simulink model "ControlLoopSim"  (R2018b)
settings: Solver=FixedStepAuto  StartTime=0.0  StopTime=Tsim  FixedStep=Ts  RelTol=1e-3
values from neighbouring files (symbols this model uses):
  Ts = 0.01    [simulation.m]    (also in simulationKoop.m)
  x0 = [80/3.6; 0; -5/180*pi]    [simulation.m]    (also in simulationKoop.m = [60/3.6; 0; -5/180*pi])
undefined symbols (not defined in the file or in its folder): nRef, nSignal, reference, steering
settings Model: Creator=Marko  LastModifiedBy=Marko

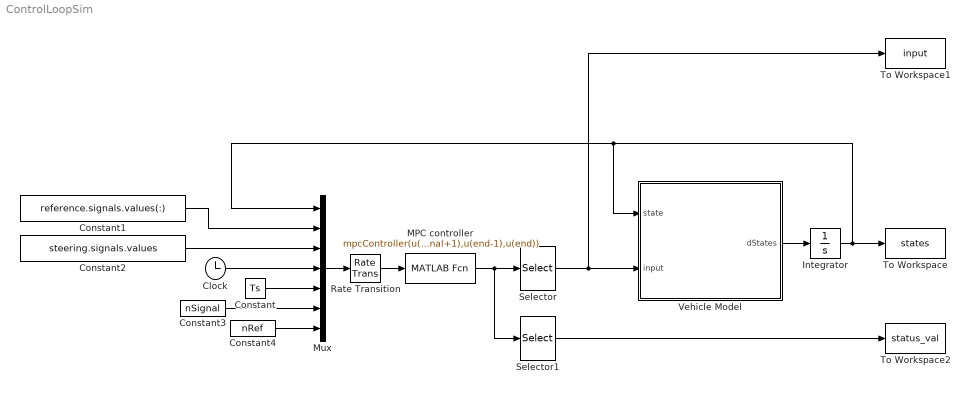
== system ControlLoopSim ==
  Clock : Clock
  Constant : Constant  Value=Ts
  Constant1 : Constant  Value=reference.signals.values(:)  SampleTime=Ts
  Constant2 : Constant  Value=steering.signals.values  SampleTime=Ts
  Constant3 : Constant  Value=nSignal
  Constant4 : Constant  Value=nRef
  Integrator : Integrator  InitialCondition=x0
  MPC controller : MATLABFcn  MATLABFcn=mpcController(u(1:3), u(4:4+nSignal*nRef-1), u(4+nSignal*nRef:4+nSignal*nRef+nSignal-1), u(4+nSignal*nRef+nSignal),u(4+nSignal*nRef+nSignal+1),u(end-1),u(end))  OutputDimensions=3 + 1
  Mux : Mux  Inputs=7
  Rate Transition : RateTransition  OutPortSampleTime=Ts
  Selector : Selector  InputPortWidth=4  IndexOptions=Index vector (dialog)  Indices=[1 2 3]  OutputSizes=1
  Selector1 : Selector  InputPortWidth=4  IndexOptions=Index vector (dialog)  Indices=4  OutputSizes=1
  To Workspace : ToWorkspace  VariableName=states  SaveFormat=Structure With Time  SampleTime=Ts
  To Workspace1 : ToWorkspace  VariableName=input  SaveFormat=Structure With Time  SampleTime=Ts
  To Workspace2 : ToWorkspace  VariableName=status_val  SaveFormat=Structure With Time  SampleTime=Ts
  Vehicle Model : MATLAB Function  TreatAsAtomicUnit=on
  wires:
  Vehicle Model/1(dStates) -> Integrator/1
  Integrator/1 -> To Workspace/1, Mux/1, Vehicle Model/1(state)
  MPC controller/1 -> Selector/1, Selector1/1
  Mux/1 -> Rate Transition/1
  Selector1/1 -> To Workspace2/1
  Selector/1 -> To Workspace1/1, Vehicle Model/2(input)
  Rate Transition/1 -> MPC controller/1
  Constant/1 -> Mux/5
  Clock/1 -> Mux/4
  Constant1/1 -> Mux/2
  Constant2/1 -> Mux/3
  Constant3/1 -> Mux/6
  Constant4/1 -> Mux/7

== matlab function ControlLoopSim/Vehicle Model ==
  data: state input; dStates output; input input
function dStates  = BicycleModel(state,input)

% Extract states
vx = state(1);
vy = state(2);
yawRate = state(3);

% Extract inputs
deltaF = input(1);
sF = input(2);
sR = input(3);

% Load parameters
vehicle = LoadVehicleParameters();

% Vehicle parameters
a = vehicle.a;
b = vehicle.b;
m = vehicle.Mass;
I = vehicle.Izz;

% Air drag parameters
cw = vehicle.cw;
rho = vehicle.rho;
Aw = vehicle.Aw;

% Tyre parameters
Cxf = vehicle.Cxf;
Cyf = vehicle.Cyf;
Cxr = vehicle.Cxr;
Cyr = vehicle.Cyr;

% Lateral velocities
vyf = vy + a*yawRate;
vyr = vy - b*yawRate;
% Longitudinal velocities
vxf = vx;
vxr = vx;

% TYRE VELOCITIES
% Cornering velocities
vcf = vyf*cos(deltaF) - vxf*sin(deltaF);
vcr = vyr;
% Longitudinal velocities
vlf = vyf*sin(deltaF) + vxf*cos(deltaF);
vlr = vxr;

% TYRE SLIP ANGLES
alpha_f = atan2(vcf,vlf);
alpha_r = atan2(vcr,vlr);

% Longitudinal and cornering forces
Flf = Cxf*sF;
Flr = Cxr*sR;
Fcf = -Cyf*alpha_f;
Fcr = -Cyr*alpha_r;

% AXLE FORCES
% Lateral forces
Fyf = Flf*sin(deltaF) + Fcf*cos(deltaF);
Fyr = Fcr;
% Longitudinal forces
Fxf = Flf*cos(deltaF) - Fcf*sin(deltaF);
Fxr = Flr;

dVx = 1/m * (m*yawRate*vy - 0.5*cw*rho*Aw*sqrt(vx^2+vy^2)*vx + Fxf + Fxr);
dVy = 1/m * (-m*yawRate*vx - 0.5*cw*rho*Aw*sqrt(vx^2+vy^2)*vy + Fyf + Fyr);
dYawRate = 1/I * (Fyf*a - Fyr*b);

dStates = [dVx; dVy; dYawRate];

end
